simulink model "ASMC_without_sensor_noise_simulink"  (R2023b)
settings: Solver=VariableStepAuto  StartTime=0.0  StopTime=30  RelTol=1e-3
values from neighbouring files (symbols this model uses):
  A = 0.4668    [ASMC_with_sensor_noise_matlab.m]    (also in ASMC_without_sensor_noise_matlab.m; FL_matlab.m = [0 1 0 0; 0 0 1 0; 0 0 0 1; 0 0 0 0])
  c1 = C(1)    [ASMC_with_sensor_noise_matlab.m]    (also in ASMC_without_sensor_noise_matlab.m)
  c2 = C(2)    [ASMC_with_sensor_noise_matlab.m]    (also in ASMC_without_sensor_noise_matlab.m)
  c3 = C(3)    [ASMC_with_sensor_noise_matlab.m]    (also in ASMC_without_sensor_noise_matlab.m)
  c4 = C(4)    [ASMC_with_sensor_noise_matlab.m]    (also in ASMC_without_sensor_noise_matlab.m)
  c5 = C(5)    [ASMC_with_sensor_noise_matlab.m]    (also in ASMC_without_sensor_noise_matlab.m)
  c6 = C(6)    [ASMC_with_sensor_noise_matlab.m]    (also in ASMC_without_sensor_noise_matlab.m)
  g = 9.81    [ASMC_with_sensor_noise_matlab.m]    (also in ASMC_without_sensor_noise_matlab.m; FL_matlab.m)
  k1 = K(1,1)    [ASMC_with_sensor_noise_matlab.m]    (also in ASMC_without_sensor_noise_matlab.m; FL_matlab.m = K(1))
  k2 = K(2,2)    [ASMC_with_sensor_noise_matlab.m]    (also in ASMC_without_sensor_noise_matlab.m; FL_matlab.m = K(2))
  k3 = K(3,3)    [ASMC_with_sensor_noise_matlab.m]    (also in ASMC_without_sensor_noise_matlab.m; FL_matlab.m = K(3))
  k4 = K(4,4)    [ASMC_with_sensor_noise_matlab.m]    (also in ASMC_without_sensor_noise_matlab.m; FL_matlab.m = K(4))
  k5 = K(5,5)    [ASMC_with_sensor_noise_matlab.m]    (also in ASMC_without_sensor_noise_matlab.m)
  k6 = K(6,6)    [ASMC_with_sensor_noise_matlab.m]    (also in ASMC_without_sensor_noise_matlab.m)
  kd = -3    [ASMC_with_sensor_noise_matlab.m]    (also in ASMC_without_sensor_noise_matlab.m)
  ki = -3    [ASMC_with_sensor_noise_matlab.m]    (also in ASMC_without_sensor_noise_matlab.m)
  kp = -5    [ASMC_with_sensor_noise_matlab.m]    (also in ASMC_without_sensor_noise_matlab.m)
  l = 1    [ASMC_with_sensor_noise_matlab.m]    (also in ASMC_without_sensor_noise_matlab.m; FL_matlab.m)
  phi_0 = pi/6    (= 0.523598775598)    [ASMC_with_sensor_noise_matlab.m]    (also in ASMC_without_sensor_noise_matlab.m; FL_matlab.m)
  psi_0 = pi/6    (= 0.523598775598)    [ASMC_with_sensor_noise_matlab.m]    (also in ASMC_without_sensor_noise_matlab.m; FL_matlab.m)
  psi_d = 0    [ASMC_with_sensor_noise_matlab.m]    (also in ASMC_without_sensor_noise_matlab.m; FL_matlab.m)
  theta_0 = pi/6    (= 0.523598775598)    [ASMC_with_sensor_noise_matlab.m]    (also in ASMC_without_sensor_noise_matlab.m; FL_matlab.m)
  x_0 = 10    [ASMC_with_sensor_noise_matlab.m]    (also in ASMC_without_sensor_noise_matlab.m; FL_matlab.m)
  x_d1 = 20    [ASMC_with_sensor_noise_matlab.m]    (also in ASMC_without_sensor_noise_matlab.m; FL_matlab.m)
  x_d2 = 0    [ASMC_with_sensor_noise_matlab.m]    (also in ASMC_without_sensor_noise_matlab.m; FL_matlab.m)
  y_0 = 10    [ASMC_with_sensor_noise_matlab.m]    (also in ASMC_without_sensor_noise_matlab.m; FL_matlab.m)
  y_d1 = -10    [ASMC_with_sensor_noise_matlab.m]    (also in ASMC_without_sensor_noise_matlab.m; FL_matlab.m)
  y_d2 = 0    [ASMC_with_sensor_noise_matlab.m]    (also in ASMC_without_sensor_noise_matlab.m; FL_matlab.m)
  z0 = 2    [ASMC_with_sensor_noise_matlab.m]    (also in ASMC_without_sensor_noise_matlab.m)
  z_0 = 20    [ASMC_with_sensor_noise_matlab.m]    (also in ASMC_without_sensor_noise_matlab.m; FL_matlab.m)
  z_d1 = 10    [ASMC_with_sensor_noise_matlab.m]    (also in ASMC_without_sensor_noise_matlab.m; FL_matlab.m)
  z_d2 = 0    [ASMC_with_sensor_noise_matlab.m]    (also in ASMC_without_sensor_noise_matlab.m; FL_matlab.m)
libraries: slpidlib x6
settings Model: Creator=Kong Youngkyoung  LastModifiedBy=Kong Youngkyoung

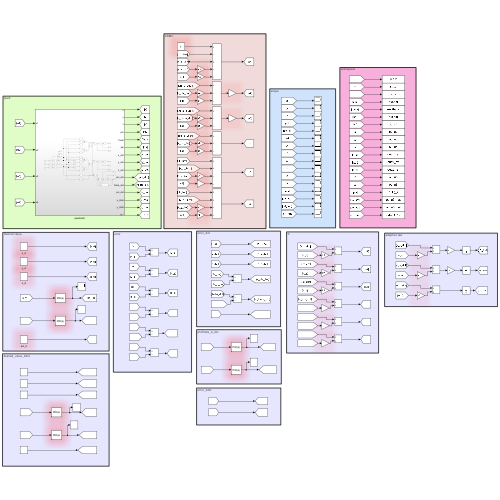
[thumbnail: Simulink's stored preview of the top-level diagram]
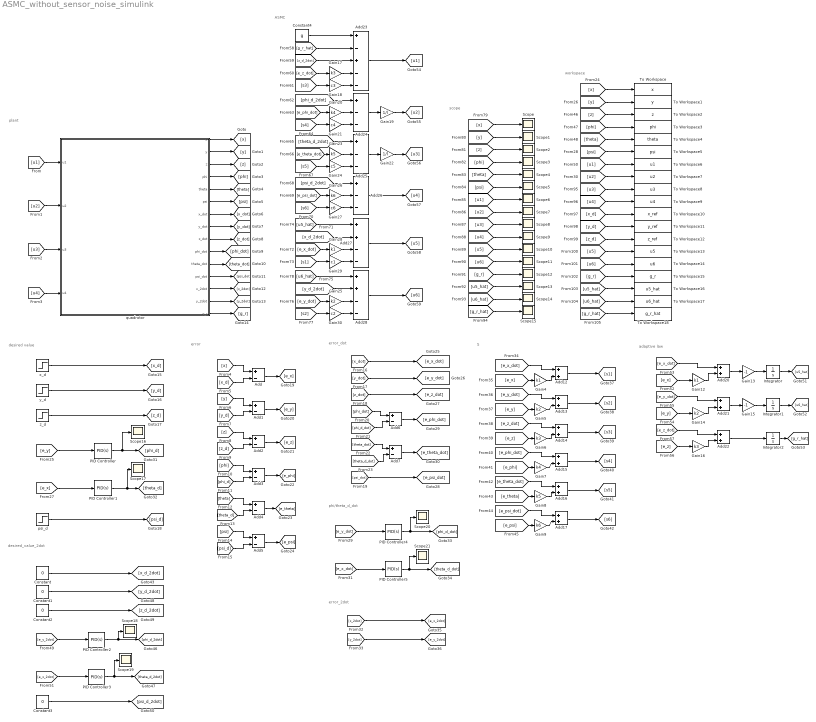
== system ASMC_without_sensor_noise_simulink ==
  note: scope
  note: ASMC
  note: adaptive law
  note: desired_value_2dot
  note: S
  note: error_2dot
  note: phi/theta_d_dot
  note: error_dot
  note: error
  note: desired value
  note: plant
  note: workspace
  Add{,1..7} (8 alike) : Sum  Inputs=+-
  Add{12..17,20..22} (9 alike) : Sum
  Add23 : Sum  Inputs=+-+--
  Add24 : Sum  Inputs=+--
  Add25 : Sum  Inputs=+--
  Add26 : Sum  Inputs=+--
  Add27 : Sum  Inputs=++--
  Add28 : Sum  Inputs=++--
  Constant{,1..3} (4 alike) : Constant  Value=0
  Constant4 : Constant  Value=g
  Gain12 : Gain  Gain=k1
  Gain13 : Gain  Gain=-1
  Gain14 : Gain  Gain=k2
  Gain15 : Gain  Gain=-1
  Gain16 : Gain  Gain=k3
  Gain17 : Gain  Gain=k3
  Gain18 : Gain  Gain=c3
  Gain19 : Gain  Gain=1/l
  Gain20 : Gain  Gain=k4
  Gain21 : Gain  Gain=c4
  Gain22 : Gain  Gain=1/l
  Gain23 : Gain  Gain=k5
  Gain24 : Gain  Gain=c5
  Gain25 : Gain  Gain=k2
  Gain26 : Gain  Gain=k6
  Gain27 : Gain  Gain=c6
  Gain28 : Gain  Gain=k1
  Gain29 : Gain  Gain=c1
  Gain30 : Gain  Gain=c2
  Gain4 : Gain  Gain=k1
  Gain5 : Gain  Gain=k2
  Gain6 : Gain  Gain=k3
  Gain7 : Gain  Gain=k4
  Gain8 : Gain  Gain=k5
  Gain9 : Gain  Gain=k6
  Integrator : Integrator
  Integrator1 : Integrator
  Integrator2 : Integrator
  PID Controller{,1..5} (6 alike) : slpidlib/PID Controller  Controller=PID  Form=Parallel  TimeDomain=Continuous-time  UseExternalTs=off  SampleTime=-1  IntegratorMethod=Forward Euler  FilterMethod=Forward Euler  ControllerParametersSource=internal  P=kp  I=ki  UseKiTs=off  D=kd  N=100  UseFilter=on  TunerSelectOption=Transfer Function Based (PID Tuner App)  InitialConditionSource=internal  InitialConditionForIntegrator=0  InitialConditionForFilter=0  DifferentiatorICPrevScaledInput=0  ExternalReset=none  TrackingMode=off  Kt=1  LimitOutput=off  SatLimitsSource=internal  UpperSaturationLimit=inf  LowerSaturationLimit=-inf  LinearizeAsGain=on  AntiWindupMode=none  Kb=1  LimitIntegrator=off  UpperIntegratorSaturationLimit=inf  LowerIntegratorSaturationLimit=-inf  POutMin=[]  POutMax=[]  IOutMin=[]  IOutMax=[]  DOutMin=[]  DOutMax=[]  NOutMin=[]  NOutMax=[]  SumOutMin=[]  SumOutMax=[]  SaturationOutMin=[]  SaturationOutMax=[]  PParamMin=[]  PParamMax=[]  IParamMin=[]  IParamMax=[]  DParamMin=[]  DParamMax=[]  NParamMin=[]  NParamMax=[]  KbParamMin=[]  KbParamMax=[]  KtParamMin=[]  KtParamMax=[]  KbOutMin=[]  KbOutMax=[]  KtOutMin=[]  KtOutMax=[]  IntegratorOutMin=[]  IntegratorOutMax=[]  FilterOutMin=[]  FilterOutMax=[]  SumI1OutMin=[]  SumI1OutMax=[]  SumI2OutMin=[]  SumI2OutMax=[]  SumI3OutMin=[]  SumI3OutMax=[]  SumI4OutMin=[]  SumI4OutMax=[]  SumDOutMin=[]  SumDOutMax=[]  DifferentiatorOutMin=[]  DifferentiatorOutMax=[]  FilterDiffOutCoefMin=[]  FilterDiffOutCoefMax=[]  ReciprocalOutMin=[]  ReciprocalOutMax=[]  SumDenOutMin=[]  SumDenOutMax=[]  SumNumOutMin=[]  SumNumOutMax=[]  DivideOutMin=[]  DivideOutMax=[]  UdiffTsProdOutMin=[]  UdiffTsProdOutMax=[]  NTsProdOutMin=[]  NTsProdOutMax=[]  UintegralTsProdOutMin=[]  UintegralTsProdOutMax=[]  UngainTsProdOutMin=[]  UngainTsProdOutMax=[]  ClampingZeroOutDataTypeStr=Inherit: Inherit via back propagation  ClampingZeroOutMin=[]  ClampingZeroOutMax=[]  FilterDenConstantOutDataTypeStr=Inherit: Inherit via back propagation  FilterDenConstantOutMin=[]  FilterDenConstantOutMax=[]  PCopyOutDataTypeStr=Inherit: Inherit via back propagation  PCopyOutMin=[]  PCopyOutMax=[]  NCopyOutDataTypeStr=Inherit: Inherit via back propagation  NCopyOutMin=[]  NCopyOutMax=[]  IntegratorContinuousStateAttributes=''  IntegratorStateMustResolveToSignalObject=off  IntegratorRTWStateStorageClass=Auto  FilterContinuousStateAttributes=''  FilterStateMustResolveToSignalObject=off  FilterRTWStateStorageClass=Auto  ParallelPVariant=InternalParameters  IdealPVariant=Disabled  IVariant=InternalParameters  DVariant=InternalParameters  IntegratorVariant=Continuous  SatVariant=Disabled  AWVariant=Passthrough  PCopyVariant=Disabled  TRVariant=Disabled  FdbkBlocksVariant=Forward  IdealPFdbkVariant=Disabled  SatFdbkVariant=Disabled  DerivativeFilterVariant=ContFilter  NVariant=InternalParameters  NCopyVariant=Disabled  FilterICVariant=InternalICsFilter  IntegratorICVariant=InternalICs  ExternalResetVariant=Disabled  TRSumVariant=Passthrough  SumFdbkVariant=Disabled  SumVariant=Sum_PID  TsampFilterVariant=InternalTs  TsampNgainVariant=Passthrough  TsampIntegralVariant=Disabled_SignalSpec  ExternalSaturationOutDataTypeStr=Inherit: Same as second input
  Scope{,1..21} (22 alike) : Scope
  To Workspace : ToWorkspace  VariableName=x  SaveFormat=Timeseries  SampleTime=-1
  To Workspace1 : ToWorkspace  VariableName=y  SaveFormat=Timeseries  SampleTime=-1
  To Workspace10 : ToWorkspace  VariableName=x_ref  SaveFormat=Timeseries  SampleTime=-1
  To Workspace11 : ToWorkspace  VariableName=y_ref  SaveFormat=Timeseries  SampleTime=-1
  To Workspace12 : ToWorkspace  VariableName=z_ref  SaveFormat=Timeseries  SampleTime=-1
  To Workspace13 : ToWorkspace  VariableName=u5  SaveFormat=Timeseries  SampleTime=-1
  To Workspace14 : ToWorkspace  VariableName=u6  SaveFormat=Timeseries  SampleTime=-1
  To Workspace15 : ToWorkspace  VariableName=g_r  SaveFormat=Timeseries  SampleTime=-1
  To Workspace16 : ToWorkspace  VariableName=u5_hat  SaveFormat=Timeseries  SampleTime=-1
  To Workspace17 : ToWorkspace  VariableName=u6_hat  SaveFormat=Timeseries  SampleTime=-1
  To Workspace18 : ToWorkspace  VariableName=g_r_hat  SaveFormat=Timeseries  SampleTime=-1
  To Workspace2 : ToWorkspace  VariableName=z  SaveFormat=Timeseries  SampleTime=-1
  To Workspace3 : ToWorkspace  VariableName=phi  SaveFormat=Timeseries  SampleTime=-1
  To Workspace4 : ToWorkspace  VariableName=theta  SaveFormat=Timeseries  SampleTime=-1
  To Workspace5 : ToWorkspace  VariableName=psi  SaveFormat=Timeseries  SampleTime=-1
  To Workspace6 : ToWorkspace  VariableName=u1  SaveFormat=Timeseries  SampleTime=-1
  To Workspace7 : ToWorkspace  VariableName=u2  SaveFormat=Timeseries  SampleTime=-1
  To Workspace8 : ToWorkspace  VariableName=u3  SaveFormat=Timeseries  SampleTime=-1
  To Workspace9 : ToWorkspace  VariableName=u4  SaveFormat=Timeseries  SampleTime=-1
  psi_d : Step  Time=15  Before=psi_d  After=psi_d  SampleTime=0
  quadrotor : Subsystem
  x_d : Step  Time=15  Before=x_d1  After=x_d2  SampleTime=0
  y_d : Step  Time=15  Before=y_d1  After=y_d2  SampleTime=0
  z_d : Step  Time=15  Before=z_d1  After=z_d2  SampleTime=0
  wires:
  quadrotor/1(x) -> [x]
  quadrotor/2(y) -> [y]
  quadrotor/3(z) -> [z]
  quadrotor/4(phi) -> [phi]
  quadrotor/5(theta) -> [theta]
  quadrotor/6(psi) -> [psi]
  quadrotor/7(x_dot) -> [x_dot]
  quadrotor/8(y_dot) -> [y_dot]
  quadrotor/10(phi_dot) -> [phi_dot]
  quadrotor/9(z_dot) -> [z_dot]
  quadrotor/11(theta_dot) -> [theta_dot]
  quadrotor/12(psi_dot) -> [psi_dot]
  quadrotor/13(x_2dot) -> [x_2dot]
  quadrotor/14(y_2dot) -> [y_2dot]
  quadrotor/15(g_r) -> [g_r]
  [u1] -> quadrotor/1(u1)
  [u2] -> quadrotor/2(u2)
  [u3] -> quadrotor/3(u3)
  [u4] -> quadrotor/4(u4)
  x_d/1 -> [x_d]
  y_d/1 -> [y_d]
  z_d/1 -> [z_d]
  psi_d/1 -> [psi_d]
  [x] -> Add/1
  [x_d] -> Add/2
  Add/1 -> [e_x]
  [y] -> Add1/1
  [y_d] -> Add1/2
  Add1/1 -> [e_y]
  [z] -> Add2/1
  [z_d] -> Add2/2
  Add2/1 -> [e_z]
  [phi] -> Add3/1
  [phi_d] -> Add3/2
  Add3/1 -> [e_phi]
  [theta] -> Add4/1
  [theta_d] -> Add4/2
  Add4/1 -> [e_theta]
  [psi] -> Add5/1
  [psi_d] -> Add5/2
  Add5/1 -> [e_psi]
  [x_dot] -> [e_x_dot]
  [y_dot] -> [e_y_dot]
  [z_dot] -> [e_z_dot]
  [psi_dot] -> [e_psi_dot]
  [phi_dot] -> Add6/1
  [phi_d_dot] -> Add6/2
  Add6/1 -> [e_phi_dot]
  [theta_d_dot] -> Add7/2
  [theta_dot] -> Add7/1
  Add7/1 -> [e_theta_dot]
  [e_y] -> PID Controller/1
  [x_2dot] -> [e_x_2dot]
  [y_2dot] -> [e_y_2dot]
  Gain4/1 -> Add12/2
  [e_x_dot] -> Add12/1
  Gain5/1 -> Add13/2
  [e_y_dot] -> Add13/1
  [e_y] -> Gain5/1
  Gain6/1 -> Add14/2
  [e_z_dot] -> Add14/1
  [e_z] -> Gain6/1
  Gain7/1 -> Add15/2
  [e_phi_dot] -> Add15/1
  [e_phi] -> Gain7/1
  Gain8/1 -> Add16/2
  [e_theta_dot] -> Add16/1
  [e_theta] -> Gain8/1
  Gain9/1 -> Add17/2
  [e_psi_dot] -> Add17/1
  [e_psi] -> Gain9/1
  Constant/1 -> [x_d_2dot]
  Constant1/1 -> [y_d_2dot]
  Constant3/1 -> [psi_d_2dot]
  Constant2/1 -> [z_d_2dot]
  [e_x] -> Gain12/1
  Gain12/1 -> Add20/2
  [e_x_dot] -> Add20/1
  Add20/1 -> Gain13/1
  Gain13/1 -> Integrator/1
  Integrator/1 -> [u5_hat]
  [e_y] -> Gain14/1
  Gain15/1 -> Integrator1/1
  Add21/1 -> Gain15/1
  Gain14/1 -> Add21/2
  [e_y_dot] -> Add21/1
  Integrator1/1 -> [u6_hat]
  [e_z] -> Gain16/1
  Add22/1 -> Integrator2/1
  Gain16/1 -> Add22/2
  [e_z_dot] -> Add22/1
  Integrator2/1 -> [g_r_hat]
  Constant4/1 -> Add23/1
  [g_r_hat] -> Add23/2
  [e_z_dot] -> Gain17/1
  Gain17/1 -> Add23/4
  [z_d_2dot] -> Add23/3
  [s3] -> Gain18/1
  Gain18/1 -> Add23/5
  Add23/1 -> [u1]
  Add24/1 -> Gain19/1
  Gain19/1 -> [u2]
  [s4] -> Gain21/1
  [e_phi_dot] -> Gain20/1
  [phi_d_2dot] -> Add24/1
  Gain20/1 -> Add24/2
  Gain21/1 -> Add24/3
  Gain22/1 -> [u3]
  [theta_d_2dot] -> Add25/1
  Gain24/1 -> Add25/3
  [e_theta_dot] -> Gain23/1
  Gain23/1 -> Add25/2
  Add25/1 -> Gain22/1
  [s5] -> Gain24/1
  Add26/1 -> [u4]
  [psi_d_2dot] -> Add26/1
  Gain27/1 -> Add26/3
  [e_psi_dot] -> Gain26/1
  Gain26/1 -> Add26/2
  [s6] -> Gain27/1
  Add27/1 -> [u5]
  [e_x_dot] -> Gain28/1
  [s1] -> Gain29/1
  [u5_hat] -> Add27/1
  [x_d_2dot] -> Add27/2
  Gain28/1 -> Add27/3
  Gain29/1 -> Add27/4
  [e_y_dot] -> Gain25/1
  Gain30/1 -> Add28/4
  [s2] -> Gain30/1
  Add28/1 -> [u6]
  Gain25/1 -> Add28/3
  [u6_hat] -> Add28/1
  [y_d_2dot] -> Add28/2
  [x] -> Scope/1
  [y] -> Scope1/1
  [z] -> Scope2/1
  [phi] -> Scope3/1
  [theta] -> Scope4/1
  [psi] -> Scope5/1
  [u1] -> Scope6/1
  [u2] -> Scope7/1
  [u3] -> Scope8/1
  [u4] -> Scope9/1
  [u5] -> Scope10/1
  [u6] -> Scope11/1
  [g_r] -> Scope12/1
  [u5_hat] -> Scope13/1
  [u6_hat] -> Scope14/1
  [g_r_hat] -> Scope15/1
  [e_x] -> Gain4/1
  Add12/1 -> [s1]
  Add13/1 -> [s2]
  Add14/1 -> [s3]
  Add15/1 -> [s4]
  Add16/1 -> [s5]
  Add17/1 -> [s6]
  PID Controller/1 -> Scope16/1, [phi_d]
  [e_x] -> PID Controller1/1
  PID Controller1/1 -> Scope17/1, [theta_d]
  [e_y_2dot] -> PID Controller2/1
  PID Controller2/1 -> Scope18/1, [phi_d_2dot]
  [e_x_2dot] -> PID Controller3/1
  PID Controller3/1 -> Scope19/1, [theta_d_2dot]
  [e_y_dot] -> PID Controller4/1
  PID Controller4/1 -> Scope20/1, [phi_d_dot]
  [e_x_dot] -> PID Controller5/1
  PID Controller5/1 -> Scope21/1, [theta_d_dot]
  [x] -> To Workspace/1
  [theta] -> To Workspace4/1
  [z_d] -> To Workspace12/1
  [u4] -> To Workspace9/1
  [y] -> To Workspace1/1
  [y_d] -> To Workspace11/1
  [u3] -> To Workspace8/1
  [u1] -> To Workspace6/1
  [z] -> To Workspace2/1
  [u2] -> To Workspace7/1
  [psi] -> To Workspace5/1
  [phi] -> To Workspace3/1
  [x_d] -> To Workspace10/1
  [u5] -> To Workspace13/1
  [u6] -> To Workspace14/1
  [g_r] -> To Workspace15/1
  [u5_hat] -> To Workspace16/1
  [u6_hat] -> To Workspace17/1
  [g_r_hat] -> To Workspace18/1

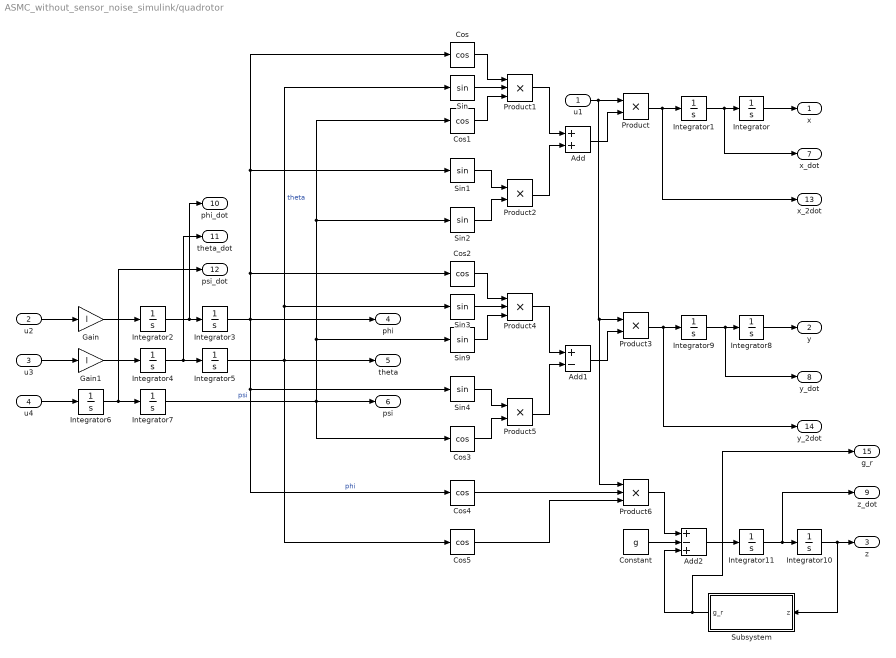
== system ASMC_without_sensor_noise_simulink/quadrotor ==
  u1 : Inport
  u2 : Inport  Port=2
  u3 : Inport  Port=3
  u4 : Inport  Port=4
  Add : Sum
  Add1 : Sum  Inputs=+-
  Add2 : Sum  Inputs=+-+
  Constant : Constant  Value=g
  Cos{,1..5} (6 alike) : Trigonometry  Operator=cos
  Gain : Gain  Gain=l
  Gain1 : Gain  Gain=l
  Integrator : Integrator  InitialCondition=x_0
  Integrator{1..2,4,6,9,11} (6 alike) : Integrator
  Integrator10 : Integrator  InitialCondition=z_0
  Integrator3 : Integrator  InitialCondition=phi_0
  Integrator5 : Integrator  InitialCondition=theta_0
  Integrator7 : Integrator  InitialCondition=psi_0
  Integrator8 : Integrator  InitialCondition=y_0
  Product{,2..3,5} (4 alike) : Product
  Product1 : Product  Inputs=3
  Product4 : Product  Inputs=3
  Product6 : Product  Inputs=3
  Sin{,1..4,9} (6 alike) : Trigonometry
  Subsystem : Subsystem
  x : Outport
  y : Outport  Port=2
  z : Outport  Port=3
  phi : Outport  Port=4
  theta : Outport  Port=5
  psi : Outport  Port=6
  x_dot : Outport  Port=7
  y_dot : Outport  Port=8
  z_dot : Outport  Port=9
  phi_dot : Outport  Port=10
  theta_dot : Outport  Port=11
  psi_dot : Outport  Port=12
  x_2dot : Outport  Port=13
  y_2dot : Outport  Port=14
  g_r : Outport  Port=15
  wires:
  Integrator/1 -> x/1
  Integrator1/1 -> x_dot/1, Integrator/1
  Product/1 -> x_2dot/1, Integrator1/1
  u1/1 -> Product/1, Product6/1, Product3/1
  Add/1 -> Product/2
  Product1/1 -> Add/1
  Product2/1 -> Add/2
  Cos/1 -> Product1/1
  Sin/1 -> Product1/2
  Cos1/1 -> Product1/3
  Sin2/1 -> Product2/2
  Sin1/1 -> Product2/1
  u2/1 -> Gain/1
  u3/1 -> Gain1/1
  Gain/1 -> Integrator2/1
  Integrator2/1 -> phi_dot/1, Integrator3/1
  Integrator3/1 -> phi/1, Sin4/1, Cos4/1, Cos2/1, Cos/1, Sin1/1  "phi"
  Integrator5/1 -> Cos5/1, Sin3/1, Sin/1, theta/1  "theta"
  Gain1/1 -> Integrator4/1
  Integrator4/1 -> theta_dot/1, Integrator5/1
  Integrator7/1 -> Cos3/1, Sin9/1, Sin2/1, Cos1/1, psi/1  "psi"
  u4/1 -> Integrator6/1
  Integrator6/1 -> psi_dot/1, Integrator7/1
  Cos3/1 -> Product5/2
  Product5/1 -> Add1/2
  Product3/1 -> y_2dot/1, Integrator9/1
  Product4/1 -> Add1/1
  Cos2/1 -> Product4/1
  Sin3/1 -> Product4/2
  Sin9/1 -> Product4/3
  Integrator9/1 -> y_dot/1, Integrator8/1
  Sin4/1 -> Product5/1
  Add1/1 -> Product3/2
  Integrator8/1 -> y/1
  Integrator11/1 -> z_dot/1, Integrator10/1
  Integrator10/1 -> Subsystem/1(z), z/1
  Product6/1 -> Add2/1
  Constant/1 -> Add2/2
  Cos4/1 -> Product6/2
  Cos5/1 -> Product6/3
  Subsystem/1(g_r) -> g_r/1, Add2/3
  Add2/1 -> Integrator11/1

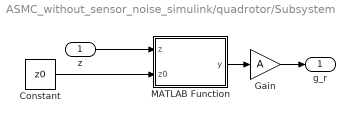
== system ASMC_without_sensor_noise_simulink/quadrotor/Subsystem ==
  z : Inport
  Constant : Constant  Value=z0
  Gain : Gain  Gain=A
  MATLAB Function : MATLAB Function  TreatAsAtomicUnit=on
  g_r : Outport
  wires:
  Gain/1 -> g_r/1
  MATLAB Function/1(y) -> Gain/1
  Constant/1 -> MATLAB Function/2(z0)
  z/1 -> MATLAB Function/1(z)

== matlab function ASMC_without_sensor_noise_simulink/quadrotor/Subsystem/MATLAB Function ==
  data: z input; y output; z0 input
function y = fcn(z, z0)

z_cg = z;
if z<=z0 && z>0
    y = (1/(z+z_cg)^2)-(1/(z0+z_cg)^2);
else
    y=0;
end
